simulink model "Simulation_rate_limited_PID"  (R2015a)
settings: Solver=FixedStepDiscrete  StartTime=0.0  StopTime=tf  FixedStep=delta_t  RelTol=1e-3
values from neighbouring files (symbols this model uses):
  delta_t = 0.001    [Constants.m]
  omega_b_0 = [0;0;0]    [Constants.m]
  psi_0 = [0;0;0;0]    [Constants.m]
  psi_max = max_rpm/60*2*pi    (= 575.958653158)    [Constants.m]
undefined symbols (not defined in the file or in its folder): q_initial
settings Model: Creator=Kerianne  LastModifiedBy=Kerianne
settings DataIOCC: SaveFormat=Structure
settings OptimizationCC: InlineParams=on  ExpressionDepthLimit=2147483647
settings DebuggingCC: UnderspecifiedInitializationDetection=Classic  MergeDetectMultiDrivingBlocksExec=none  SolverPrmCheckMsg=warning  StateNameClashWarn=warning

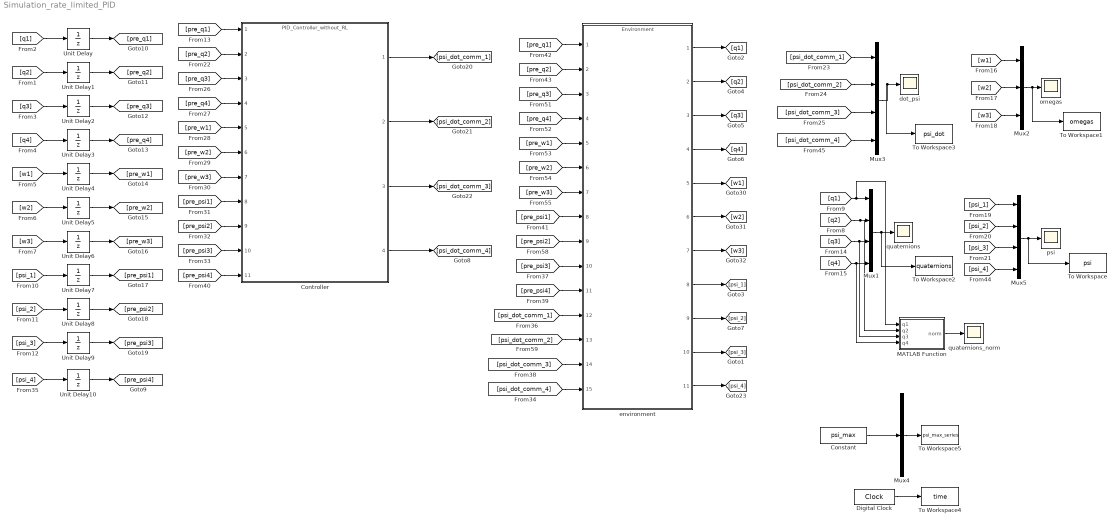
== system Simulation_rate_limited_PID ==
  Constant : Constant  Value=psi_max
  Controller : ModelReference  ModelNameDialog=PID_Controller_without_RL.slx  SimulationMode=Normal  ModelReferenceVersion=1.18  CopyOfModelName=PID_Controller_without_RL.slx  DefaultDataLogging=on
  Digital Clock : DigitalClock  SampleTime=delta_t
  MATLAB Function : MATLAB Function  TreatAsAtomicUnit=on
  Mux1 : Mux
  Mux2 : Mux  Inputs=3
  Mux3 : Mux
  Mux4 : Mux  Inputs=1
  Mux5 : Mux
  To Workspace : ToWorkspace  VariableName=psi  SaveFormat=Timeseries  SampleTime=-1
  To Workspace1 : ToWorkspace  VariableName=omegas  SaveFormat=Timeseries  SampleTime=-1
  To Workspace2 : ToWorkspace  VariableName=quaternions  SaveFormat=Timeseries  SampleTime=-1
  To Workspace3 : ToWorkspace  VariableName=psi_dot  SaveFormat=Timeseries  SampleTime=-1
  To Workspace4 : ToWorkspace  VariableName=time  SaveFormat=Timeseries  SampleTime=-1
  To Workspace5 : ToWorkspace  VariableName=psi_max_series  SaveFormat=Timeseries  SampleTime=-1
  Unit Delay : UnitDelay  InitialCondition=q_initial(1)  SampleTime=-1
  Unit Delay1 : UnitDelay  InitialCondition=q_initial(2)  SampleTime=-1
  Unit Delay10 : UnitDelay  InitialCondition=psi_0(3)  SampleTime=-1
  Unit Delay2 : UnitDelay  InitialCondition=q_initial(3)  SampleTime=-1
  Unit Delay3 : UnitDelay  InitialCondition=q_initial(4)  SampleTime=-1
  Unit Delay4 : UnitDelay  InitialCondition=omega_b_0(1)  SampleTime=-1
  Unit Delay5 : UnitDelay  InitialCondition=omega_b_0(2)  SampleTime=-1
  Unit Delay6 : UnitDelay  InitialCondition=omega_b_0(3)  SampleTime=-1
  Unit Delay7 : UnitDelay  InitialCondition=psi_0(1)  SampleTime=-1
  Unit Delay8 : UnitDelay  InitialCondition=psi_0(2)  SampleTime=-1
  Unit Delay9 : UnitDelay  InitialCondition=psi_0(3)  SampleTime=-1
  dot_psi : Scope
      settings: SaveName=ScopeData2
  environment : ModelReference  ModelNameDialog=Environment  SimulationMode=Normal  ModelReferenceVersion=1.13  CopyOfModelName=Environment  DefaultDataLogging=on
  omegas : Scope
  psi : Scope
      settings: SaveName=ScopeData3
  quaternions : Scope
  quaternions_norm : Scope
      settings: SaveName=ScopeData4
  wires:
  [pre_q1] -> Controller/1
  [pre_q2] -> Controller/2
  [pre_q3] -> Controller/3
  [pre_q4] -> Controller/4
  [pre_w1] -> Controller/5
  [pre_w2] -> Controller/6
  [pre_w3] -> Controller/7
  [pre_psi1] -> Controller/8
  [pre_psi2] -> Controller/9
  [pre_psi3] -> Controller/10
  [q1] -> Unit Delay/1
  [q2] -> Unit Delay1/1
  [q3] -> Unit Delay2/1
  [q4] -> Unit Delay3/1
  [w1] -> Unit Delay4/1
  [w2] -> Unit Delay5/1
  [w3] -> Unit Delay6/1
  [psi_1] -> Unit Delay7/1
  [psi_3] -> Unit Delay9/1
  [psi_2] -> Unit Delay8/1
  Unit Delay/1 -> [pre_q1]
  Unit Delay1/1 -> [pre_q2]
  Unit Delay2/1 -> [pre_q3]
  Unit Delay3/1 -> [pre_q4]
  Unit Delay4/1 -> [pre_w1]
  Unit Delay5/1 -> [pre_w2]
  Unit Delay6/1 -> [pre_w3]
  Unit Delay7/1 -> [pre_psi1]
  Unit Delay8/1 -> [pre_psi2]
  Unit Delay9/1 -> [pre_psi3]
  Controller/1 -> [psi_dot_comm_1]
  Controller/2 -> [psi_dot_comm_2]
  Controller/3 -> [psi_dot_comm_3]
  [q4] -> MATLAB Function/4(q4), Mux1/4
  [q2] -> MATLAB Function/2(q2), Mux1/2
  [q1] -> MATLAB Function/1(q1), Mux1/1
  Mux2/1 -> To Workspace1/1, omegas/1
  [w3] -> Mux2/3
  [w2] -> Mux2/2
  [w1] -> Mux2/1
  Mux3/1 -> To Workspace3/1, dot_psi/1
  Mux5/1 -> To Workspace/1, psi/1
  [psi_3] -> Mux5/3
  [psi_2] -> Mux5/2
  [psi_1] -> Mux5/1
  [psi_dot_comm_1] -> Mux3/1
  [psi_dot_comm_3] -> Mux3/3
  [psi_dot_comm_2] -> Mux3/2
  Mux1/1 -> To Workspace2/1, quaternions/1
  [pre_psi1] -> environment/8
  environment/10 -> [psi_3]
  environment/9 -> [psi_2]
  environment/8 -> [psi_1]
  [pre_psi2] -> environment/9
  [pre_psi3] -> environment/10
  [pre_w3] -> environment/7
  [pre_w2] -> environment/6
  [pre_w1] -> environment/5
  [pre_q4] -> environment/4
  [pre_q3] -> environment/3
  [pre_q2] -> environment/2
  [pre_q1] -> environment/1
  environment/1 -> [q1]
  environment/2 -> [q2]
  environment/3 -> [q3]
  environment/4 -> [q4]
  environment/5 -> [w1]
  environment/6 -> [w2]
  environment/7 -> [w3]
  Controller/4 -> [psi_dot_comm_4]
  [psi_4] -> Unit Delay10/1
  Unit Delay10/1 -> [pre_psi4]
  [pre_psi4] -> environment/11
  [psi_dot_comm_1] -> environment/12
  [psi_dot_comm_2] -> environment/13
  [psi_dot_comm_3] -> environment/14
  [psi_dot_comm_4] -> environment/15
  environment/11 -> [psi_4]
  [pre_psi4] -> Controller/11
  [psi_4] -> Mux5/4
  [psi_dot_comm_4] -> Mux3/4
  Digital Clock/1 -> To Workspace4/1
  Mux4/1 -> To Workspace5/1
  Constant/1 -> Mux4/1
  [q3] -> MATLAB Function/3(q3), Mux1/3
  MATLAB Function/1(norm) -> quaternions_norm/1

== matlab function Simulation_rate_limited_PID/MATLAB Function ==
  data: q1 input; norm output; q2 input; q3 input; q4 input
function norm = fcn(q1,q2,q3,q4)
%#codegen

norm = sqrt(q1^2 + q2^2+ q3^2 + q4^2);
